simulink model "http_method_post_thingspeak_demo"  (Simulink 7.3)
settings: Solver=ode3  SolverMode=SingleTasking  StartTime=0.0  StopTime=10.0  RelTol=1e-3
PreLoadFcn:
  | waijung.modelPreload; % Required for working with Waijung Blockset. Do not remove.
undefined symbols (not defined in the file): A1, A2, A7, B13, C1, C4, C5, G11, G13, HSEOSC, Link, LQFP144, ST, STM32F429ZI
libraries: simulink x11, waijung_string_manipulate x3, waijung_webserver x2, waijung_http_client_lib x2, stm32f4_adc_lib x1, stm32f4_io_lib x1, stm32f4_device_config_lib x1
CloseFcn:
  | waijung.modelClose; % Required for working with Waijung Blockset. Do not remove.
settings Model: Creator=Krisada  LastModifiedBy=Krisada
settings OptimizationCC: OptimizeModelRefInitCode=on  LifeSpan=1
settings DebuggingCC: StrictBusMsg=ErrorLevel1
settings HardwareCC: ProdEndianess=LittleEndian  ProdHWDeviceType=ARM Compatible->Cortex - M4  TargetEndianess=LittleEndian  TargetHWDeviceType=ARM Compatible->Cortex - M4
settings RTWCC: SystemTargetFile=stm32f4.tlc  GenerateMakefile=off  TemplateMakefile=ert_default_tmf  Description=STM32F4 Target  ProcessScript=stm32f4_make_rtw_hook
settings CodeAppCC: IgnoreCustomStorageClasses=off
settings STFCustomTargetCC: ModelReferenceCompliant=off  CombineOutputUpdateFcns=on  ERTCustomFileBanners=on  SupportContinuousTime=off  SupportNonInlinedSFcns=off  SystemTargetFile=stm32f4.tlc
settings ERTTargetCC: MultiwordLength=2048  ModelReferenceCompliant=off  ParMdlRefBuildCompliant=off  CompOptLevelCompliant=off  ERTFirstTimeCompliant=off  ModelStepFunctionPrototypeControlCompliant=off  CPPClassGenCompliant=off  InlinedParameterPlacement=NonHierarchical  ERTSrcFileBannerTemplate=stm32f4_code_template.cgt  ERTHdrFileBannerTemplate=stm32f4_code_template.cgt  ERTDataSrcFileTemplate=stm32f4_code_template.cgt  ERTDataHdrFileTemplate=stm32f4_code_template.cgt  ERTCustomFileTemplate=stm32f4_file_process.tlc

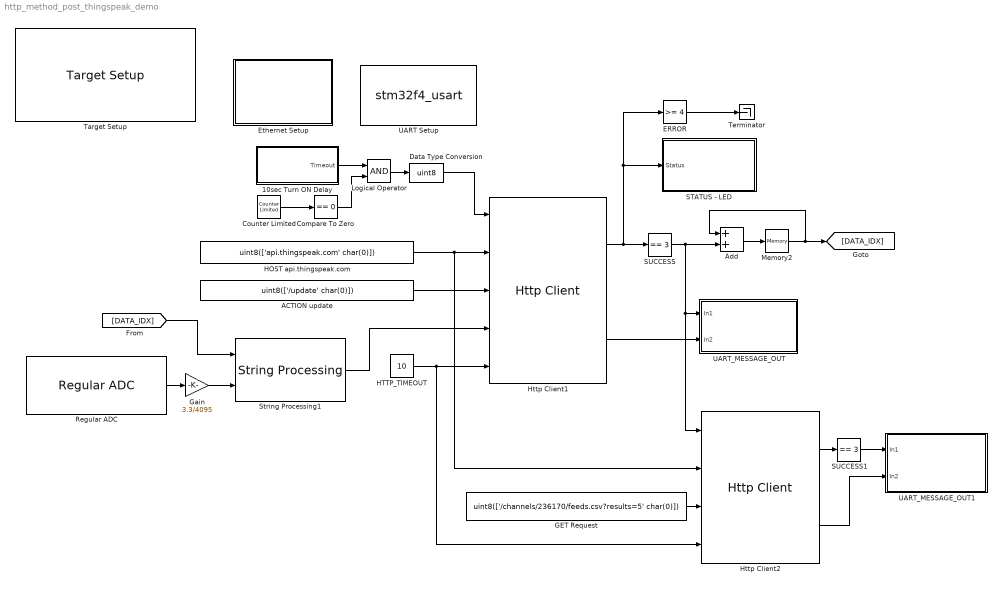
== system http_method_post_thingspeak_demo ==
  10sec Turn ON Delay : Subsystem
  ACTION update : Constant  Value=uint8(['/update' char(0)])  SampleTime=-1
  Add : Sum
  Compare To Zero : simulink/Logic and Bit Operations/Compare To Zero  SystemSampleTime=-1  relop===  LogicOutDataTypeMode=uint8
  Counter Limited : simulink/Sources/Counter Limited  SystemSampleTime=-1  uplimit=499  tsamp=-1
  Data Type Conversion : DataTypeConversion  OutDataTypeMode=uint8  OutDataTypeStr=uint8
  ERROR : simulink/Logic and Bit Operations/Compare To Constant  SystemSampleTime=-1  relop=>=  const=4  LogicOutDataTypeMode=uint8
  Ethernet Setup : Subsystem
  GET Request : Constant  Value=uint8(['/channels/236170/feeds.csv?results=5' char(0)])  SampleTime=-1
  Gain : Gain  Gain=3.3/4095
  HOST api.thingspeak.com : Constant  Value=uint8(['api.thingspeak.com' char(0)])  SampleTime=-1
  HTTP_TIMEOUT : Constant  Value=10  OutDataTypeMode=uint32  OutDataTypeStr=uint32  SampleTime=-1
  Http Client1 : waijung_http_client_lib/Http Client  conf=HttpPOST  contenttype='application/x-www-form-urlencoded'  httpresponse=on  httpresponsesize=1024  beginpattern=''  terminatorpattern=''  portpinstr=0  sampletime=0.01  blockid=HttpClient1  inputporttype=[-1 3 3 3 7]  inputportwidth=[1 -1 -1 -1 1]  inputportlabel={'Trig','Host','Action','Content','Timeout(sec)'}  outputporttype=[3 3]  outputportwidth=[1 1024]  outputportlabel={'Status','Response'}  compat=0  optionstring="[\"on\",\"application/x-www-form-urlencoded\"]"  stringparam1=0  stringparam2=0
  Http Client2 : waijung_http_client_lib/Http Client  conf=HttpGET  contenttype='application/x-www-form-urlencoded'  httpresponse=on  httpresponsesize=1024  beginpattern=''  terminatorpattern=''  portpinstr=0  sampletime=0.01  blockid=HttpClient2  inputporttype=[-1 3 3 7]  inputportwidth=[1 -1 -1 1]  inputportlabel={'Trig','Host','Request','Timeout(sec)'}  outputporttype=[3 3]  outputportwidth=[1 1024]  outputportlabel={'Status','Response'}  compat=0  optionstring="[\"on\",\"application/x-www-form-urlencoded\"]"  stringparam1=0  stringparam2=0
  Logical Operator : Logic  AllPortsSameDT=off  OutDataTypeMode=boolean  OutDataTypeStr=boolean
  Memory2 : Memory  InheritSampleTime=on  LinearizeMemory=on  LinearizeAsDelay=on
  Regular ADC : stm32f4_adc_lib/Regular ADC  adcmodule=1  outputdatatype=Single  prescaler=2  prescalerstr=ADC_Prescaler_Div2  chsamplingtime=Auto  chsamplingtimestr=ADC_SampleTime_480Cycles  read_an0=off  read_an1=off  read_an2=off  read_an3=off  read_an4=off  read_an5=off  read_an6=off  read_an7=off  read_an8=off  read_an9=on  read_an10=off  read_an11=off  read_an12=off  read_an13=off  read_an14=off  read_an15=off  read_an16=off  read_an17=off  read_an18=off  pinstr=GPIO_Pin_9  usedpinarray="[0  0  0  0  0  0  0  0  0  1  0  0  0  0  0  0  0  0  0]"  usedportidarray=[1]  usedpinidarray=[1]  usedpinidcount=1  sampletime=-1  blockid=RegularADC  enablecustomportlabel=off  cinputportlabel=0  coutputportlabel=Out1, Out2
  STATUS - LED : Subsystem
  SUCCESS : simulink/Logic and Bit Operations/Compare To Constant  SystemSampleTime=-1  relop===  const=3  LogicOutDataTypeMode=uint8
  SUCCESS1 : simulink/Logic and Bit Operations/Compare To Constant  SystemSampleTime=-1  relop===  const=3  LogicOutDataTypeMode=uint8
  String Processing1 : waijung_string_manipulate/String Processing  conf=processing  stringfunction=sprintf  stringformat='api_key=LLYHIMHACKG50HOH&field1=%u&field2=%1.2f'  begindelimiter=''  enddelimiter=''  buffersize=512  enablestatus=off  portpinstr=0  sampletime=-1  blockid=StringProcessing1  inputporttype=[-1 -1]  inputportwidth=[1 1]  inputportlabel={'%u','%f'}  outputporttype=[3]  outputportwidth=[512]  outputportlabel={'Output'}  compat=0  optionstring=[]  datatypestring="[\"uint32_t\",\"float\"]"
  Target Setup : stm32f4_device_config_lib/Target Setup  Priority=100  compiler=GNU ARM  previous_compiler=GNU ARM  mcu=STM32F429ZI (LQFP144)  mcustr=STM32F429ZI  clockconfig=HSEOSC-8MHz  system_stm32f4xx_c_path=F:\trunk\targets\stm32f4_target\stm32f4\utils\system_stm32f4xx_default\STM32F429_439xx\hseosc8mhz  showmemoryconfiguration=off  stacksize=0x2000  heapsize=0x2000  enableautocompiledownload=on  fullchiperase=off  programmerinterface=ST-Link  editctrlstr=on  compilercontrolstr=$(patsubst %, -I%, .) -mcpu=cortex-m4 -mthumb -mthumb-interwork -mfloat-abi=hard -mfpu=fpv4-sp-d16 -ffast-math -Wall -Wextra -Ofast  assemblercontrolstr=$(patsubst %, -I%, .) -mcpu=cortex-m4 -mthumb -mthumb-interwork -mfloat-abi=hard -mfpu=fpv4-sp-d16 -ffast-math -Wall -Wextra -Ofast -Wa,-amhls=$(<:.s=.lst) -D__STACK_SIZE=$(STACK_SIZE) -D__HEAP_SIZE=$(HEAP_SIZE)  linkercontrolstr=-T$(LD_SCRIPT) -g -Wl,-Map=$(MAP),--cref,--no-warn-mismatch -mcpu=cortex-m4 -mthumb -mthumb-interwork -mfloat-abi=hard -mfpu=fpv4-sp-d16 -specs=nosys.specs  runafterdownload=on  execprofile=None  profileruart=3  profilerbaud=500000  profilertxpin=D8  profilerinitstr=0.01,180000000,1800000,500000,0  manualsetsampletime=off  sampletime=0.01  blockid=TargetSetup  systickreloadvalue=1800000  hseval=8000000  lastprofileruart=3  hclk=180000000  flashorigin=0x8000000  flashlength=2048k  ramorigin=0x20000000  ramlength=192k  useextram=off
  Terminator : Terminator
  UART Setup : S-Function  Priority=1  FunctionName=stm32f4_usart  Parameters=configuration,uartmodule,transfer,baudrate,inputtype,outputtype,confstr,binheaderarray,binterminatorarray,asciiheader,asciiterminator,bindatalength,packetmode,varname,sampletime,sampletimestr,blockid  EnableBusSupport=off  mask(stm32f4_usart){configuration=Setup, uartmodule=3, baudrate=115200, databits=8, parity=No, stopbit=1, remaptxpin=D8, remaprxpin=D9, flowcontrol=None, remapctspin=Not used, remaprtspin=Not used, advanceoptions=on, rxbuffersize=512, txbuffersize=1024, transfer=Blocking, packetmode=Ascii, binheader='7E 7E', binterminator='03 03', porttype_double=1, porttype_single=0, porttype_int8=1, porttype_uint8=0, porttype_int16=0, porttype_uint16=0, porttype_int32=0, porttype_uint32=0, asciiformat='%d,%f', rx_asciiterminator=CR (0x0D - "\\\\r"), tx_asciiterminator=CR (0x0D - "\\\\r"), storagename=<empty>, varname=, inputtype=[0], outputtype=[0], binheaderarray=[0], binterminatorarray=[0], bindatalength=0, asciiheader='', asciiterminator=[0], sampletime=-1, sampletimestr=0.01, blockid=UARTSetup, confstr=[ "dummy", "1", "D", "8", "1", "D", "9", "0", "*", "*", "0", "*", "*", "1", "4", "3", "1", "4", "1", "1024", "512", "1", "3", "115200", "8", "No", "1", "None", "USART3"], lastmodule=3}
      mask prompts: uartmodule "UART Module"; baudrate "Baud rate (bps)"; databits "Data bits"; stopbit "Stop bit"; remaptxpin "Tx Pin"; remaprxpin "Rx Pin"; flowcontrol "Hardware flow control"; remapctspin "HW Flow control, CTS Pin"; remaprtspin "HW Flow control, RTS Pin"; advanceoptions "Advance options"; rxbuffersize "Rx buffer size (bytes)"; txbuffersize "Tx buffer size (bytes)"; packetmode "Packet mode"; binheader "Binary header (example: '7E 7E')"; binterminator "Binary terminator (example: '03 03')"; porttype_double "Number of data port, type DOUBLE"; porttype_single "Number of data port, type SINGLE"; porttype_int8 "Number of data port, type INT8"; porttype_uint8 "Number of data port, type UINT8"; porttype_int16 "Number of data port, type INT16"; porttype_uint16 "Number of data port, type UINT16"; porttype_int32 "Number of data port, type INT32"; porttype_uint32 "Number of data port, type UINT32"; asciiformat "Ascii format"; rx_asciiterminator "End of packet"; tx_asciiterminator "End of packet"; storagename "Buffer"; varname "Var name"; inputtype "Input data type"; outputtype "Output data type"; binheaderarray "Binary header"; binterminatorarray "Binary terminator"; bindatalength "Binary data length"; asciiheader "Ascii header (printf format)"; asciiterminator "Ascii terminator"; sampletime "Sample time (sec)"; sampletimestr "Compiled sample time (sec) in string"; confstr "Configuration string"; lastmodule "Last module selected"
      mask help:
      | Default STM32F4DISCOVERY + aMG F4 Connect 2 + aMG USB Converter N2 settings use
      |
      | USART3, Tx D8, Rx D9 and USB Serial Converter A.
      mask init:
      | stm32f4_usart_callback('init');
      mask Help: web(fullfile(waijungdocroot,'stm32f4_usart_setup.htm'), '-browser')
      mask StyleString: popup(Setup|Tx|Rx),popup(1|2|3|4|5|6),edit,popup(8),popup(No|Odd|Even),popup(0.5|1|1.5|2),popup(Not used|B10|C10|D8),popup(Not used|B11|C11|D9),popup(None|RTS|CTS|RTS/CTS),popup(Not used|B13|D11),popup(Not used|B14|D12),checkbox,popup(16|32|64|128|256|512|1024|2048),popup(16|32|64|128|256|512|1024|2048),popup(Blocking|Non-Blocking),popup(Ascii|Binary|String Buffer),edit,edit,edit,edit,edit,edit,edit,edit,edit,edit,edit,popup(CR (0x0D - "\\\\r")|LF (0x0A - "\\\\n")|CRLF (0x0D 0x0A - "\\\\r\\\\n")),popup(CR (0x0D - "\\\\r")|LF (0x0A - "\\\\n")|CRLF (0x0D 0x0A - "\\\\r\\\\n")|None),popup(<empty>),edit,edit,edit,edit,edit,edit,edit,edit,edit,edit,edit,edit,edit
      mask CallbackString: stm32f4_usart_callback('configuration');|stm32f4_usart_callback('uartmodule');|stm32f4_usart_callback('baudrate');||||||stm32f4_usart_callback('flowcontrol');|||stm32f4_usart_callback('advanceoptions');|||stm32f4_usart_callback('transfer');|stm32f4_usart_callback('packetmode');|stm32f4_usart_callback('binheader');|stm32f4_usart_callback('binterminator');|stm32f4_usart_callback('porttype');|stm32f4_usart_callback('porttype');|stm32f4_usart_callback('porttype');|stm32f4_usart_callback('porttype');|stm32f4_usart_callback('porttype');|stm32f4_usart_callback('porttype');|stm32f4_usart_callback('porttype');|stm32f4_usart_callback('porttype');|stm32f4_usart_callback('asciiformat');|stm32f4_usart_callback('rx_asciiterminator');|stm32f4_usart_callback('tx_asciiterminator');|stm32f4_usart_callback('storagename');|stm32f4_usart_callback('varname');||||||||stm32f4_usart_callback('sampletime');|stm32f4_usart_callback('sampletimestr');|stm32f4_usart_callback('blockid');||
      mask Display: text(0.5, 0.5, 'Module: USART3_Setup\nBaud (Bps): 115200\nDMA Buffer: 1024/512\nTx/Rx Pin: D8/D9','ver','middle','hor','center');
  UART_MESSAGE_OUT : Subsystem
  UART_MESSAGE_OUT1 : Subsystem
  wires:
  Counter Limited/1 -> Compare To Zero/1
  HOST api.thingspeak.com/1 -> Http Client2/2, Http Client1/2
  HTTP_TIMEOUT/1 -> Http Client2/4, Http Client1/5
  SUCCESS/1 -> Add/2, UART_MESSAGE_OUT/1(In1), Http Client2/1
  String Processing1/1 -> Http Client1/4
  Regular ADC/1 -> Gain/1
  Add/1 -> Memory2/1
  Memory2/1 -> Add/1, [DATA_IDX]
  Http Client1/1 -> SUCCESS/1, STATUS - LED/1(Status), ERROR/1
  Http Client1/2 -> UART_MESSAGE_OUT/2(In2)
  Gain/1 -> String Processing1/2
  [DATA_IDX] -> String Processing1/1
  10sec Turn ON Delay/1(Timeout) -> Logical Operator/1
  Compare To Zero/1 -> Logical Operator/2
  Logical Operator/1 -> Data Type Conversion/1
  ERROR/1 -> Terminator/1
  Data Type Conversion/1 -> Http Client1/1
  ACTION update/1 -> Http Client1/3
  GET Request/1 -> Http Client2/3
  Http Client2/1 -> SUCCESS1/1
  SUCCESS1/1 -> UART_MESSAGE_OUT1/1(In1)
  Http Client2/2 -> UART_MESSAGE_OUT1/2(In2)

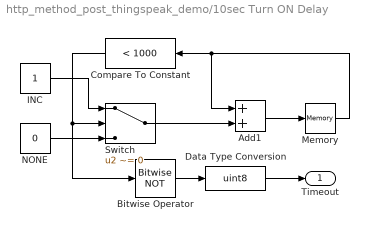
== system http_method_post_thingspeak_demo/10sec Turn ON Delay ==
  Add1 : Sum
  Bitwise Operator : simulink/Logic and Bit Operations/Bitwise Operator  logicop=NOT  UseBitMask=off  BitMask=bin2dec('11011001')  BitMaskRealWorld=Stored Integer
  Compare To Constant : simulink/Logic and Bit Operations/Compare To Constant  SystemSampleTime=-1  relop=<  const=1000  LogicOutDataTypeMode=uint8
  Data Type Conversion : DataTypeConversion  OutDataTypeMode=uint8  OutDataTypeStr=uint8
  INC : Constant  OutDataTypeMode=int32  OutDataTypeStr=int32  SampleTime=-1
  Memory : Memory  InheritSampleTime=on  LinearizeMemory=on  LinearizeAsDelay=on
  NONE : Constant  Value=0  OutDataTypeMode=int32  OutDataTypeStr=int32  SampleTime=-1
  Switch : Switch  Criteria=u2 ~= 0
  Timeout : Outport
  wires:
  Memory/1 -> Add1/1, Compare To Constant/1
  INC/1 -> Switch/1
  Switch/1 -> Add1/2
  NONE/1 -> Switch/3
  Add1/1 -> Memory/1
  Compare To Constant/1 -> Bitwise Operator/1, Switch/2
  Bitwise Operator/1 -> Data Type Conversion/1
  Data Type Conversion/1 -> Timeout/1

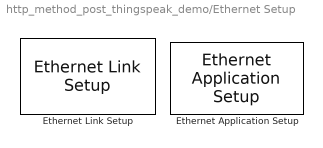
== system http_method_post_thingspeak_demo/Ethernet Setup ==
  Ethernet Application Setup : waijung_webserver/Ethernet Application Setup  conf=Setup  ipaddress=192.168.1.42  netmask=255.255.255.0  gateway=192.168.1.1  macaddress=02-00-00-00-00-00  dhcp=off  timerscaler=250  portpinstr=0  sampletime=-1  blockid=EthernetSetupEthernetApplicationSetup  inputporttype=[]  inputportwidth=[]  inputportlabel={}  outputporttype=[]  outputportwidth=[]  outputportlabel={}  compat=0  optionstring="[\"Dummy\",\"192\",\"168\",\"1\",\"42\",\"255\",\"255\",\"255\",\"0\",\"192\",\"168\",\"1\",\"1\",\"02\",\"00\",\"00\",\"00\",\"00\",\"00\",\"off\",\"250\"]"
  Ethernet Link Setup : waijung_webserver/Ethernet Link Setup  conf=Setup  interfacepin=Manual  chipaddress=0  wj_interfacetype=RMII  pin_mdio=A2  pin_mdc=C1  pin_pps=Not used  pin_crs=A0  pin_col=A3  pin_dv=A7  pin_rxclk=A1  pin_rxer=B10  pin_rxd0=C4  pin_rxd1=C5  pin_rxd2=B0  pin_rxd3=B1  pin_txclk=C3  pin_txen=G11  pin_txd0=G13  pin_txd1=B13  pin_txd2=C2  pin_txd3=E2  portpinstr=A1,A2,A7,G11,G13,B13,C1,C4,C5,  sampletime=-1  blockid=EthernetSetupEthernetLinkSetup  inputporttype=[]  inputportwidth=[]  inputportlabel={}  outputporttype=[]  outputportwidth=[]  outputportlabel={}  compat=0  optionstring="[\"xxx\",\"on\",\"on\",\"on\",\"off\",\"off\",\"off\",\"on\",\"off\",\"off\",\"off\",\"on\",\"on\",\"off\",\"on\",\"off\",\"off\",\"off\",\"off\",\"off\",\"on\",\"on\",\"on\",\"on\",\"off\",\"off\",\"on\",\"on\",\"A\",\"0\",\"A\",\"1\",\"A\",\"2\",\"A\",\"3\",\"A\",\"7\",\"B\",\"0\",\"B\",\"1\",\"N\",\"ot used\",\"E\",\"2\",\"B\",\"10\",\"G\",\"11\",\"G\",\"13\",\"B\",\"13\",\"C\",\"1\",\"C\",\"2\",\"C\",\"3\",\"C\",\"4\",\"C\",\"5\",\"RMII\",\"0\"]"

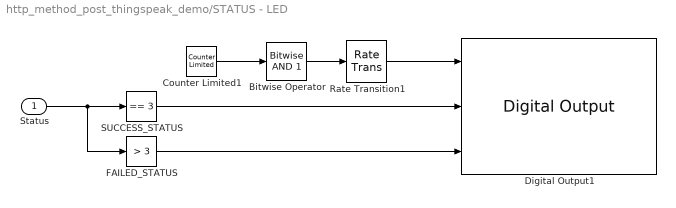
== system http_method_post_thingspeak_demo/STATUS - LED ==
  Status : Inport
  Bitwise Operator : simulink/Logic and Bit Operations/Bitwise Operator  logicop=AND  UseBitMask=on  BitMask=1  BitMaskRealWorld=Stored Integer
  Counter Limited1 : simulink/Sources/Counter Limited  SystemSampleTime=-1  uplimit=99  tsamp=0.1
  Digital Output1 : stm32f4_io_lib/Digital Output  use_bitband=on  port=B  speed=100  porttype=Push Pull  porttypestr=PP  use_pin0=on  use_pin1=off  use_pin2=off  use_pin3=off  use_pin4=off  use_pin5=off  use_pin6=off  use_pin7=on  use_pin8=off  use_pin9=off  use_pin10=off  use_pin11=off  use_pin12=off  use_pin13=off  use_pin14=on  use_pin15=off  pinstr=GPIO_Pin_0 | GPIO_Pin_7 | GPIO_Pin_14  usedpinarray="[1  0  0  0  0  0  0  1  0  0  0  0  0  0  1  0]"  bitbandingstr=|  sampletime=-1  sampletimestr=0.01  blockid=STATUSLEDDigitalOutput1  enablecustomportlabel=off  globalinit=off  cinputportlabel=In1, In2  coutputportlabel=0
      | #define STATUSLEDDigitalOutput1_B0 Peripheral_BB(GPIOB->ODR, 0)  /* Output pin */
      | #define STATUSLEDDigitalOutput1_B7 Peripheral_BB(GPIOB->ODR, 7)  /* Output pin */
      | #define STATUSLEDDigitalOutput1_B14 Peripheral_BB(GPIOB->ODR, 14)  /* Output pin */
  FAILED_STATUS : simulink/Logic and Bit Operations/Compare To Constant  SystemSampleTime=-1  relop=>  const=3  LogicOutDataTypeMode=uint8
  Rate Transition1 : RateTransition
  SUCCESS_STATUS : simulink/Logic and Bit Operations/Compare To Constant  SystemSampleTime=-1  relop===  const=3  LogicOutDataTypeMode=uint8
  wires:
  FAILED_STATUS/1 -> Digital Output1/3
  Rate Transition1/1 -> Digital Output1/1
  SUCCESS_STATUS/1 -> Digital Output1/2
  Status/1 -> FAILED_STATUS/1, SUCCESS_STATUS/1
  Bitwise Operator/1 -> Rate Transition1/1
  Counter Limited1/1 -> Bitwise Operator/1

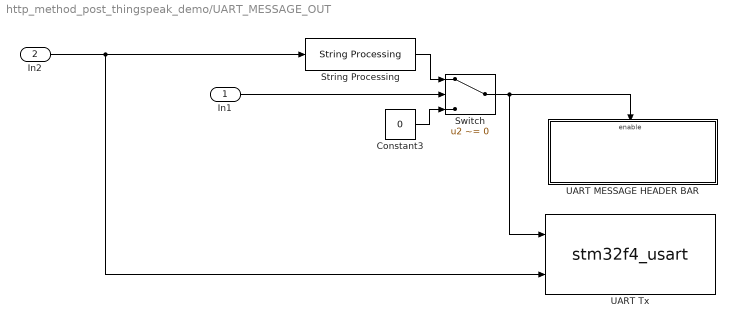
== system http_method_post_thingspeak_demo/UART_MESSAGE_OUT ==
  In1 : Inport
  In2 : Inport  Port=2
  Constant3 : Constant  Value=0  OutDataTypeMode=uint16  OutDataTypeStr=uint16  SampleTime=-1
  String Processing : waijung_string_manipulate/String Processing  conf=processing  stringfunction=strlen  stringformat='value=%d,%f'  begindelimiter=''  enddelimiter=''  buffersize=28  enablestatus=off  portpinstr=0  sampletime=-1  blockid=UART_MESSAGE_OUTStringProcessing  inputporttype=[3]  inputportwidth=[-1]  inputportlabel={'Input'}  outputporttype=[7]  outputportwidth=[1]  outputportlabel={'Length'}  compat=0  optionstring=[]  datatypestring=[]
  Switch : Switch  Criteria=u2 ~= 0
  UART MESSAGE HEADER BAR : Subsystem
  UART Tx : S-Function  Priority=1  FunctionName=stm32f4_usart  Parameters=configuration,uartmodule,transfer,baudrate,inputtype,outputtype,confstr,binheaderarray,binterminatorarray,asciiheader,asciiterminator,bindatalength,packetmode,varname,sampletime,sampletimestr,blockid  EnableBusSupport=off  mask(stm32f4_usart){configuration=Tx, uartmodule=3, baudrate=115200, databits=8, parity=No, stopbit=1, remaptxpin=Not used, remaprxpin=Not used, flowcontrol=None, remapctspin=Not used, remaprtspin=Not used, advanceoptions=off, rxbuffersize=512, txbuffersize=512, transfer=Blocking, packetmode=Raw Buffer, binheader='7E 7E', binterminator='03 03', porttype_double=1, porttype_single=0, porttype_int8=1, porttype_uint8=0, porttype_int16=0, porttype_uint16=0, porttype_int32=0, porttype_uint32=0, asciiformat='value=%d,%f', rx_asciiterminator=CR (0x0D - "\\\\r"), tx_asciiterminator=CR (0x0D - "\\\\r"), storagename=<empty>, varname=, inputtype=[2  7 262147], outputtype=[0], binheaderarray=[0], binterminatorarray=[0], bindatalength=1024, asciiheader='value=%d,%f\r\n', asciiterminator=[2 13 10], sampletime=-1, sampletimestr=0.01, blockid=UART_MESSAGE_OUTUARTTx, confstr=[ "dummy", "0", "*", "*", "0", "*", "*", "0", "*", "*", "0", "*", "*", "1", "4", "3", "1", "4", "1", "512", "512", "1", "3", "115200", "8", "No", "1", "None", "USART3"], lastmodule=1}
      mask prompts: uartmodule "UART Module"; baudrate "Baud rate (bps)"; databits "Data bits"; stopbit "Stop bit"; remaptxpin "Tx Pin"; remaprxpin "Rx Pin"; flowcontrol "Hardware flow control"; remapctspin "HW Flow control, CTS Pin"; remaprtspin "HW Flow control, RTS Pin"; advanceoptions "Advance options"; rxbuffersize "Rx buffer size (bytes)"; txbuffersize "Tx buffer size (bytes)"; packetmode "Packet mode"; binheader "Binary header (example: '7E 7E')"; binterminator "Binary terminator (example: '03 03')"; porttype_double "Number of data port, type DOUBLE"; porttype_single "Number of data port, type SINGLE"; porttype_int8 "Number of data port, type INT8"; porttype_uint8 "Number of data port, type UINT8"; porttype_int16 "Number of data port, type INT16"; porttype_uint16 "Number of data port, type UINT16"; porttype_int32 "Number of data port, type INT32"; porttype_uint32 "Number of data port, type UINT32"; asciiformat "Ascii format"; rx_asciiterminator "End of packet"; tx_asciiterminator "End of packet"; storagename "Buffer"; varname "Var name"; inputtype "Input data type"; outputtype "Output data type"; binheaderarray "Binary header"; binterminatorarray "Binary terminator"; bindatalength "Binary data length"; asciiheader "Ascii header (printf format)"; asciiterminator "Ascii terminator"; sampletime "Sample time (sec)"; sampletimestr "Compiled sample time (sec) in string"; confstr "Configuration string"; lastmodule "Last module selected"
      mask help:
      | Data type for Ascii format
      | %u, %i, %d, %o, %x: uint32
      | %e, %g, %f: single
      | %c: int8
      mask init:
      | stm32f4_usart_callback('init');
      mask Help: web(fullfile(waijungdocroot,'stm32f4_usart_tx.htm'), '-browser')
      mask StyleString: popup(Setup|Tx|Rx),popup(1|2|3|4|5|6),edit,popup(8),popup(No|Odd|Even),popup(0.5|1|1.5|2),popup(Not used|A9|B6),popup(Not used|A10|B7),popup(None|RTS|CTS|RTS/CTS),popup(Not used|A11),popup(Not used|A12),checkbox,popup(16|32|64|128|256|512|1024|2048),popup(16|32|64|128|256|512|1024|2048),popup(Blocking|Non-Blocking),popup(Ascii|Binary|Binary Vector|String Buffer|Raw Buffer),edit,edit,edit,edit,edit,edit,edit,edit,edit,edit,edit,popup(CR (0x0D - "\\\\r")|LF (0x0A - "\\\\n")|CRLF (0x0D 0x0A - "\\\\r\\\\n")),popup(CR (0x0D - "\\\\r")|LF (0x0A - "\\\\n")|CRLF (0x0D 0x0A - "\\\\r\\\\n")|None),popup(<empty>),edit,edit,edit,edit,edit,edit,edit,edit,edit,edit,edit,edit,edit
      mask CallbackString: stm32f4_usart_callback('configuration');|stm32f4_usart_callback('uartmodule');|stm32f4_usart_callback('baudrate');||||||stm32f4_usart_callback('flowcontrol');|||stm32f4_usart_callback('advanceoptions');|||stm32f4_usart_callback('transfer');|stm32f4_usart_callback('packetmode');|stm32f4_usart_callback('binheader');|stm32f4_usart_callback('binterminator');|stm32f4_usart_callback('porttype');|stm32f4_usart_callback('porttype');|stm32f4_usart_callback('porttype');|stm32f4_usart_callback('porttype');|stm32f4_usart_callback('porttype');|stm32f4_usart_callback('porttype');|stm32f4_usart_callback('porttype');|stm32f4_usart_callback('porttype');|stm32f4_usart_callback('asciiformat');|stm32f4_usart_callback('rx_asciiterminator');|stm32f4_usart_callback('tx_asciiterminator');|stm32f4_usart_callback('storagename');|stm32f4_usart_callback('varname');||||||||stm32f4_usart_callback('sampletime');|stm32f4_usart_callback('sampletimestr');|stm32f4_usart_callback('blockid');||
      mask Display: text(0.95, 0.5, 'Module: USART3_Tx\nPacket: Raw Buffer\nTransfer: Blocking\nTs (sec): 0.01','ver','middle','hor','right'); port_label('input', 1,'tx_len'); port_label('input', 2,'uint8(1024)');
  wires:
  In1/1 -> Switch/2
  String Processing/1 -> Switch/1
  Switch/1 -> UART Tx/1, UART MESSAGE HEADER BAR/Enable
  Constant3/1 -> Switch/3
  In2/1 -> UART Tx/2, String Processing/1

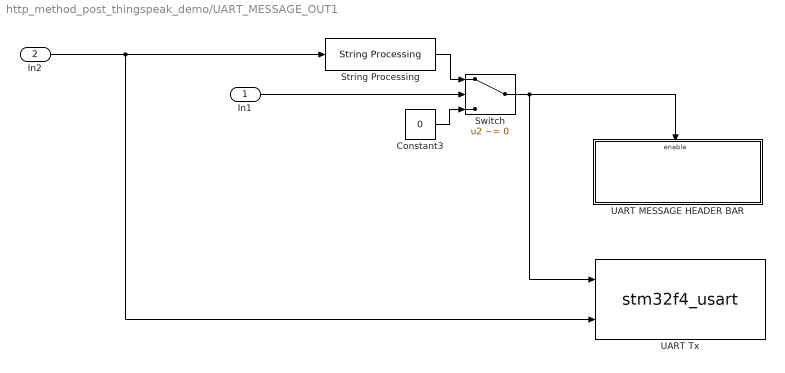
== system http_method_post_thingspeak_demo/UART_MESSAGE_OUT1 ==
  In1 : Inport
  In2 : Inport  Port=2
  Constant3 : Constant  Value=0  OutDataTypeMode=uint16  OutDataTypeStr=uint16  SampleTime=-1
  String Processing : waijung_string_manipulate/String Processing  conf=processing  stringfunction=strlen  stringformat='value=%d,%f'  begindelimiter=''  enddelimiter=''  buffersize=28  enablestatus=off  portpinstr=0  sampletime=-1  blockid=UART_MESSAGE_OUT1StringProcessing  inputporttype=[3]  inputportwidth=[-1]  inputportlabel={'Input'}  outputporttype=[7]  outputportwidth=[1]  outputportlabel={'Length'}  compat=0  optionstring=[]  datatypestring=[]
  Switch : Switch  Criteria=u2 ~= 0
  UART MESSAGE HEADER BAR : Subsystem
  UART Tx : S-Function  Priority=1  FunctionName=stm32f4_usart  Parameters=configuration,uartmodule,transfer,baudrate,inputtype,outputtype,confstr,binheaderarray,binterminatorarray,asciiheader,asciiterminator,bindatalength,packetmode,varname,sampletime,sampletimestr,blockid  EnableBusSupport=off  mask(stm32f4_usart){configuration=Tx, uartmodule=3, baudrate=115200, databits=8, parity=No, stopbit=1, remaptxpin=Not used, remaprxpin=Not used, flowcontrol=None, remapctspin=Not used, remaprtspin=Not used, advanceoptions=off, rxbuffersize=512, txbuffersize=512, transfer=Blocking, packetmode=Raw Buffer, binheader='7E 7E', binterminator='03 03', porttype_double=1, porttype_single=0, porttype_int8=1, porttype_uint8=0, porttype_int16=0, porttype_uint16=0, porttype_int32=0, porttype_uint32=0, asciiformat='value=%d,%f', rx_asciiterminator=CR (0x0D - "\\\\r"), tx_asciiterminator=CR (0x0D - "\\\\r"), storagename=<empty>, varname=, inputtype=[2  7 262147], outputtype=[0], binheaderarray=[0], binterminatorarray=[0], bindatalength=1024, asciiheader='value=%d,%f\r\n', asciiterminator=[2 13 10], sampletime=-1, sampletimestr=0.01, blockid=UART_MESSAGE_OUT1UARTTx, confstr=[ "dummy", "0", "*", "*", "0", "*", "*", "0", "*", "*", "0", "*", "*", "1", "4", "3", "1", "4", "1", "512", "512", "1", "3", "115200", "8", "No", "1", "None", "USART3"], lastmodule=1}
      mask prompts: uartmodule "UART Module"; baudrate "Baud rate (bps)"; databits "Data bits"; stopbit "Stop bit"; remaptxpin "Tx Pin"; remaprxpin "Rx Pin"; flowcontrol "Hardware flow control"; remapctspin "HW Flow control, CTS Pin"; remaprtspin "HW Flow control, RTS Pin"; advanceoptions "Advance options"; rxbuffersize "Rx buffer size (bytes)"; txbuffersize "Tx buffer size (bytes)"; packetmode "Packet mode"; binheader "Binary header (example: '7E 7E')"; binterminator "Binary terminator (example: '03 03')"; porttype_double "Number of data port, type DOUBLE"; porttype_single "Number of data port, type SINGLE"; porttype_int8 "Number of data port, type INT8"; porttype_uint8 "Number of data port, type UINT8"; porttype_int16 "Number of data port, type INT16"; porttype_uint16 "Number of data port, type UINT16"; porttype_int32 "Number of data port, type INT32"; porttype_uint32 "Number of data port, type UINT32"; asciiformat "Ascii format"; rx_asciiterminator "End of packet"; tx_asciiterminator "End of packet"; storagename "Buffer"; varname "Var name"; inputtype "Input data type"; outputtype "Output data type"; binheaderarray "Binary header"; binterminatorarray "Binary terminator"; bindatalength "Binary data length"; asciiheader "Ascii header (printf format)"; asciiterminator "Ascii terminator"; sampletime "Sample time (sec)"; sampletimestr "Compiled sample time (sec) in string"; confstr "Configuration string"; lastmodule "Last module selected"
      mask help:
      | Data type for Ascii format
      | %u, %i, %d, %o, %x: uint32
      | %e, %g, %f: single
      | %c: int8
      mask init:
      | stm32f4_usart_callback('init');
      mask Help: web(fullfile(waijungdocroot,'stm32f4_usart_tx.htm'), '-browser')
      mask StyleString: popup(Setup|Tx|Rx),popup(1|2|3|4|5|6),edit,popup(8),popup(No|Odd|Even),popup(0.5|1|1.5|2),popup(Not used|A9|B6),popup(Not used|A10|B7),popup(None|RTS|CTS|RTS/CTS),popup(Not used|A11),popup(Not used|A12),checkbox,popup(16|32|64|128|256|512|1024|2048),popup(16|32|64|128|256|512|1024|2048),popup(Blocking|Non-Blocking),popup(Ascii|Binary|Binary Vector|String Buffer|Raw Buffer),edit,edit,edit,edit,edit,edit,edit,edit,edit,edit,edit,popup(CR (0x0D - "\\\\r")|LF (0x0A - "\\\\n")|CRLF (0x0D 0x0A - "\\\\r\\\\n")),popup(CR (0x0D - "\\\\r")|LF (0x0A - "\\\\n")|CRLF (0x0D 0x0A - "\\\\r\\\\n")|None),popup(<empty>),edit,edit,edit,edit,edit,edit,edit,edit,edit,edit,edit,edit,edit
      mask CallbackString: stm32f4_usart_callback('configuration');|stm32f4_usart_callback('uartmodule');|stm32f4_usart_callback('baudrate');||||||stm32f4_usart_callback('flowcontrol');|||stm32f4_usart_callback('advanceoptions');|||stm32f4_usart_callback('transfer');|stm32f4_usart_callback('packetmode');|stm32f4_usart_callback('binheader');|stm32f4_usart_callback('binterminator');|stm32f4_usart_callback('porttype');|stm32f4_usart_callback('porttype');|stm32f4_usart_callback('porttype');|stm32f4_usart_callback('porttype');|stm32f4_usart_callback('porttype');|stm32f4_usart_callback('porttype');|stm32f4_usart_callback('porttype');|stm32f4_usart_callback('porttype');|stm32f4_usart_callback('asciiformat');|stm32f4_usart_callback('rx_asciiterminator');|stm32f4_usart_callback('tx_asciiterminator');|stm32f4_usart_callback('storagename');|stm32f4_usart_callback('varname');||||||||stm32f4_usart_callback('sampletime');|stm32f4_usart_callback('sampletimestr');|stm32f4_usart_callback('blockid');||
      mask Display: text(0.95, 0.5, 'Module: USART3_Tx\nPacket: Raw Buffer\nTransfer: Blocking\nTs (sec): 0.01','ver','middle','hor','right'); port_label('input', 1,'tx_len'); port_label('input', 2,'uint8(1024)');
  wires:
  In2/1 -> UART Tx/2, String Processing/1
  Constant3/1 -> Switch/3
  Switch/1 -> UART MESSAGE HEADER BAR/Enable, UART Tx/1
  String Processing/1 -> Switch/1
  In1/1 -> Switch/2

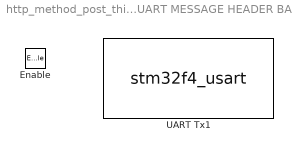
== system http_method_post_thingspeak_demo/UART_MESSAGE_OUT/UART MESSAGE HEADER BAR ==
  Enable : EnablePort
  UART Tx1 : S-Function  Priority=0  FunctionName=stm32f4_usart  Parameters=configuration,uartmodule,transfer,baudrate,inputtype,outputtype,confstr,binheaderarray,binterminatorarray,asciiheader,asciiterminator,bindatalength,packetmode,varname,sampletime,sampletimestr,blockid  EnableBusSupport=off  mask(stm32f4_usart){configuration=Tx, uartmodule=3, baudrate=115200, databits=8, parity=No, stopbit=1, remaptxpin=Not used, remaprxpin=Not used, flowcontrol=None, remapctspin=Not used, remaprtspin=Not used, advanceoptions=off, rxbuffersize=512, txbuffersize=512, transfer=Blocking, packetmode=Ascii, binheader='7E 7E', binterminator='03 03', porttype_double=1, porttype_single=0, porttype_int8=1, porttype_uint8=0, porttype_int16=0, porttype_uint16=0, porttype_int32=0, porttype_uint32=0, asciiformat='\r\n=========== POST ===========\r\n', rx_asciiterminator=CR (0x0D - "\\\\r"), tx_asciiterminator=CR (0x0D - "\\\\r"), storagename=<empty>, varname=, inputtype=[0 ], outputtype=[0], binheaderarray=[0], binterminatorarray=[0], bindatalength=0, asciiheader='\r\n=========== POST ===========\r\n\r\n', asciiterminator=[2 13 10], sampletime=-1, sampletimestr=0.01, blockid=UART_MESSAGE_OUTUARTMESSAGEHEADERBARUARTTx1, confstr=[ "dummy", "0", "*", "*", "0", "*", "*", "0", "*", "*", "0", "*", "*", "1", "4", "3", "1", "4", "1", "512", "512", "1", "3", "115200", "8", "No", "1", "None", "USART3"], lastmodule=1}
      mask prompts: uartmodule "UART Module"; baudrate "Baud rate (bps)"; databits "Data bits"; stopbit "Stop bit"; remaptxpin "Tx Pin"; remaprxpin "Rx Pin"; flowcontrol "Hardware flow control"; remapctspin "HW Flow control, CTS Pin"; remaprtspin "HW Flow control, RTS Pin"; advanceoptions "Advance options"; rxbuffersize "Rx buffer size (bytes)"; txbuffersize "Tx buffer size (bytes)"; packetmode "Packet mode"; binheader "Binary header (example: '7E 7E')"; binterminator "Binary terminator (example: '03 03')"; porttype_double "Number of data port, type DOUBLE"; porttype_single "Number of data port, type SINGLE"; porttype_int8 "Number of data port, type INT8"; porttype_uint8 "Number of data port, type UINT8"; porttype_int16 "Number of data port, type INT16"; porttype_uint16 "Number of data port, type UINT16"; porttype_int32 "Number of data port, type INT32"; porttype_uint32 "Number of data port, type UINT32"; asciiformat "Ascii format"; rx_asciiterminator "End of packet"; tx_asciiterminator "End of packet"; storagename "Buffer"; varname "Var name"; inputtype "Input data type"; outputtype "Output data type"; binheaderarray "Binary header"; binterminatorarray "Binary terminator"; bindatalength "Binary data length"; asciiheader "Ascii header (printf format)"; asciiterminator "Ascii terminator"; sampletime "Sample time (sec)"; sampletimestr "Compiled sample time (sec) in string"; confstr "Configuration string"; lastmodule "Last module selected"
      mask help:
      | Data type for Ascii format
      | %u, %i, %d, %o, %x: uint32
      | %e, %g, %f: single
      | %c: int8
      mask init:
      | stm32f4_usart_callback('init');
      mask Help: web(fullfile(waijungdocroot,'stm32f4_usart_tx.htm'), '-browser')
      mask StyleString: popup(Setup|Tx|Rx),popup(1|2|3|4|5|6),edit,popup(8),popup(No|Odd|Even),popup(0.5|1|1.5|2),popup(Not used|A9|B6),popup(Not used|A10|B7),popup(None|RTS|CTS|RTS/CTS),popup(Not used|A11),popup(Not used|A12),checkbox,popup(16|32|64|128|256|512|1024|2048),popup(16|32|64|128|256|512|1024|2048),popup(Blocking|Non-Blocking),popup(Ascii|Binary|Binary Vector|String Buffer|Raw Buffer),edit,edit,edit,edit,edit,edit,edit,edit,edit,edit,edit,popup(CR (0x0D - "\\\\r")|LF (0x0A - "\\\\n")|CRLF (0x0D 0x0A - "\\\\r\\\\n")),popup(CR (0x0D - "\\\\r")|LF (0x0A - "\\\\n")|CRLF (0x0D 0x0A - "\\\\r\\\\n")|None),popup(<empty>),edit,edit,edit,edit,edit,edit,edit,edit,edit,edit,edit,edit,edit
      mask CallbackString: stm32f4_usart_callback('configuration');|stm32f4_usart_callback('uartmodule');|stm32f4_usart_callback('baudrate');||||||stm32f4_usart_callback('flowcontrol');|||stm32f4_usart_callback('advanceoptions');|||stm32f4_usart_callback('transfer');|stm32f4_usart_callback('packetmode');|stm32f4_usart_callback('binheader');|stm32f4_usart_callback('binterminator');|stm32f4_usart_callback('porttype');|stm32f4_usart_callback('porttype');|stm32f4_usart_callback('porttype');|stm32f4_usart_callback('porttype');|stm32f4_usart_callback('porttype');|stm32f4_usart_callback('porttype');|stm32f4_usart_callback('porttype');|stm32f4_usart_callback('porttype');|stm32f4_usart_callback('asciiformat');|stm32f4_usart_callback('rx_asciiterminator');|stm32f4_usart_callback('tx_asciiterminator');|stm32f4_usart_callback('storagename');|stm32f4_usart_callback('varname');||||||||stm32f4_usart_callback('sampletime');|stm32f4_usart_callback('sampletimestr');|stm32f4_usart_callback('blockid');||
      mask Display: text(0.95, 0.5, 'Module: USART3_Tx\nPacket: Ascii\nTransfer: Blocking\nTs (sec): 0.01','ver','middle','hor','right');

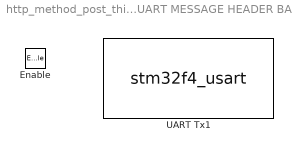
== system http_method_post_thingspeak_demo/UART_MESSAGE_OUT1/UART MESSAGE HEADER BAR ==
  Enable : EnablePort
  UART Tx1 : S-Function  Priority=0  FunctionName=stm32f4_usart  Parameters=configuration,uartmodule,transfer,baudrate,inputtype,outputtype,confstr,binheaderarray,binterminatorarray,asciiheader,asciiterminator,bindatalength,packetmode,varname,sampletime,sampletimestr,blockid  EnableBusSupport=off  mask(stm32f4_usart){configuration=Tx, uartmodule=3, baudrate=115200, databits=8, parity=No, stopbit=1, remaptxpin=Not used, remaprxpin=Not used, flowcontrol=None, remapctspin=Not used, remaprtspin=Not used, advanceoptions=off, rxbuffersize=512, txbuffersize=512, transfer=Blocking, packetmode=Ascii, binheader='7E 7E', binterminator='03 03', porttype_double=1, porttype_single=0, porttype_int8=1, porttype_uint8=0, porttype_int16=0, porttype_uint16=0, porttype_int32=0, porttype_uint32=0, asciiformat='\r\n=========== GET ===========\r\n', rx_asciiterminator=CR (0x0D - "\\\\r"), tx_asciiterminator=CR (0x0D - "\\\\r"), storagename=<empty>, varname=, inputtype=[0 ], outputtype=[0], binheaderarray=[0], binterminatorarray=[0], bindatalength=0, asciiheader='\r\n=========== GET ===========\r\n\r\n', asciiterminator=[2 13 10], sampletime=-1, sampletimestr=0.01, blockid=UART_MESSAGE_OUT1UARTMESSAGEHEADERBARUARTTx1, confstr=[ "dummy", "0", "*", "*", "0", "*", "*", "0", "*", "*", "0", "*", "*", "1", "4", "3", "1", "4", "1", "512", "512", "1", "3", "115200", "8", "No", "1", "None", "USART3"], lastmodule=1}
      mask prompts: uartmodule "UART Module"; baudrate "Baud rate (bps)"; databits "Data bits"; stopbit "Stop bit"; remaptxpin "Tx Pin"; remaprxpin "Rx Pin"; flowcontrol "Hardware flow control"; remapctspin "HW Flow control, CTS Pin"; remaprtspin "HW Flow control, RTS Pin"; advanceoptions "Advance options"; rxbuffersize "Rx buffer size (bytes)"; txbuffersize "Tx buffer size (bytes)"; packetmode "Packet mode"; binheader "Binary header (example: '7E 7E')"; binterminator "Binary terminator (example: '03 03')"; porttype_double "Number of data port, type DOUBLE"; porttype_single "Number of data port, type SINGLE"; porttype_int8 "Number of data port, type INT8"; porttype_uint8 "Number of data port, type UINT8"; porttype_int16 "Number of data port, type INT16"; porttype_uint16 "Number of data port, type UINT16"; porttype_int32 "Number of data port, type INT32"; porttype_uint32 "Number of data port, type UINT32"; asciiformat "Ascii format"; rx_asciiterminator "End of packet"; tx_asciiterminator "End of packet"; storagename "Buffer"; varname "Var name"; inputtype "Input data type"; outputtype "Output data type"; binheaderarray "Binary header"; binterminatorarray "Binary terminator"; bindatalength "Binary data length"; asciiheader "Ascii header (printf format)"; asciiterminator "Ascii terminator"; sampletime "Sample time (sec)"; sampletimestr "Compiled sample time (sec) in string"; confstr "Configuration string"; lastmodule "Last module selected"
      mask help:
      | Data type for Ascii format
      | %u, %i, %d, %o, %x: uint32
      | %e, %g, %f: single
      | %c: int8
      mask init:
      | stm32f4_usart_callback('init');
      mask Help: web(fullfile(waijungdocroot,'stm32f4_usart_tx.htm'), '-browser')
      mask StyleString: popup(Setup|Tx|Rx),popup(1|2|3|4|5|6),edit,popup(8),popup(No|Odd|Even),popup(0.5|1|1.5|2),popup(Not used|A9|B6),popup(Not used|A10|B7),popup(None|RTS|CTS|RTS/CTS),popup(Not used|A11),popup(Not used|A12),checkbox,popup(16|32|64|128|256|512|1024|2048),popup(16|32|64|128|256|512|1024|2048),popup(Blocking|Non-Blocking),popup(Ascii|Binary|Binary Vector|String Buffer|Raw Buffer),edit,edit,edit,edit,edit,edit,edit,edit,edit,edit,edit,popup(CR (0x0D - "\\\\r")|LF (0x0A - "\\\\n")|CRLF (0x0D 0x0A - "\\\\r\\\\n")),popup(CR (0x0D - "\\\\r")|LF (0x0A - "\\\\n")|CRLF (0x0D 0x0A - "\\\\r\\\\n")|None),popup(<empty>),edit,edit,edit,edit,edit,edit,edit,edit,edit,edit,edit,edit,edit
      mask CallbackString: stm32f4_usart_callback('configuration');|stm32f4_usart_callback('uartmodule');|stm32f4_usart_callback('baudrate');||||||stm32f4_usart_callback('flowcontrol');|||stm32f4_usart_callback('advanceoptions');|||stm32f4_usart_callback('transfer');|stm32f4_usart_callback('packetmode');|stm32f4_usart_callback('binheader');|stm32f4_usart_callback('binterminator');|stm32f4_usart_callback('porttype');|stm32f4_usart_callback('porttype');|stm32f4_usart_callback('porttype');|stm32f4_usart_callback('porttype');|stm32f4_usart_callback('porttype');|stm32f4_usart_callback('porttype');|stm32f4_usart_callback('porttype');|stm32f4_usart_callback('porttype');|stm32f4_usart_callback('asciiformat');|stm32f4_usart_callback('rx_asciiterminator');|stm32f4_usart_callback('tx_asciiterminator');|stm32f4_usart_callback('storagename');|stm32f4_usart_callback('varname');||||||||stm32f4_usart_callback('sampletime');|stm32f4_usart_callback('sampletimestr');|stm32f4_usart_callback('blockid');||
      mask Display: text(0.95, 0.5, 'Module: USART3_Tx\nPacket: Ascii\nTransfer: Blocking\nTs (sec): 0.01','ver','middle','hor','right');
